simulink model "a2_sim_model"  (R2023a)
settings: Solver=ode4  StartTime=0.0  StopTime=end_time  FixedStep=dt  MaxStep=0.001  RelTol=1e-3
values from neighbouring files (symbols this model uses):
  dt = 0.001    [a3_main_scipt.m]
  IC = [x_ic, theta_ic, D_x_ic, D_theta_ic]'    [a3_main_scipt.m]
  K_Dtheta = 3    [a3_main_scipt.m]
  K_Dx = 0.01    [a3_main_scipt.m]
  K_theta = 30    [a3_main_scipt.m]
  K_x = 0.01    [a3_main_scipt.m]
libraries: simulink x2
settings Model: Creator=Adam  LastModifiedBy=Adam
settings SolverCC: AlgebraicLoopSolver=TrustRegion
settings DebuggingCC: AlgebraicLoopMsg=none  UnconnectedInputMsg=warning  UnconnectedOutputMsg=warning  UnconnectedLineMsg=warning
settings ModelReferenceCC: EnableRefExpFcnMdlSchedulingChecks=on
settings RTWCC: DLArmComputeVersion=19.05

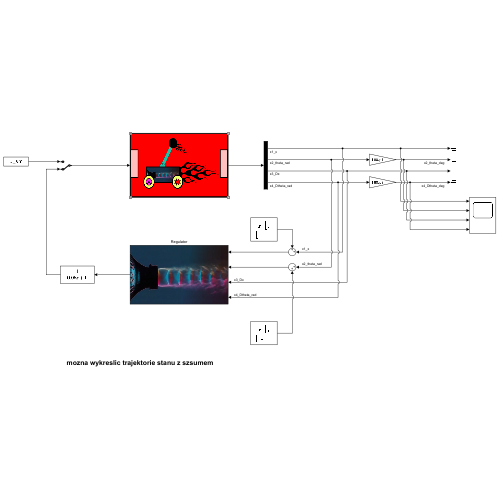
[thumbnail: Simulink's stored preview of the top-level diagram]
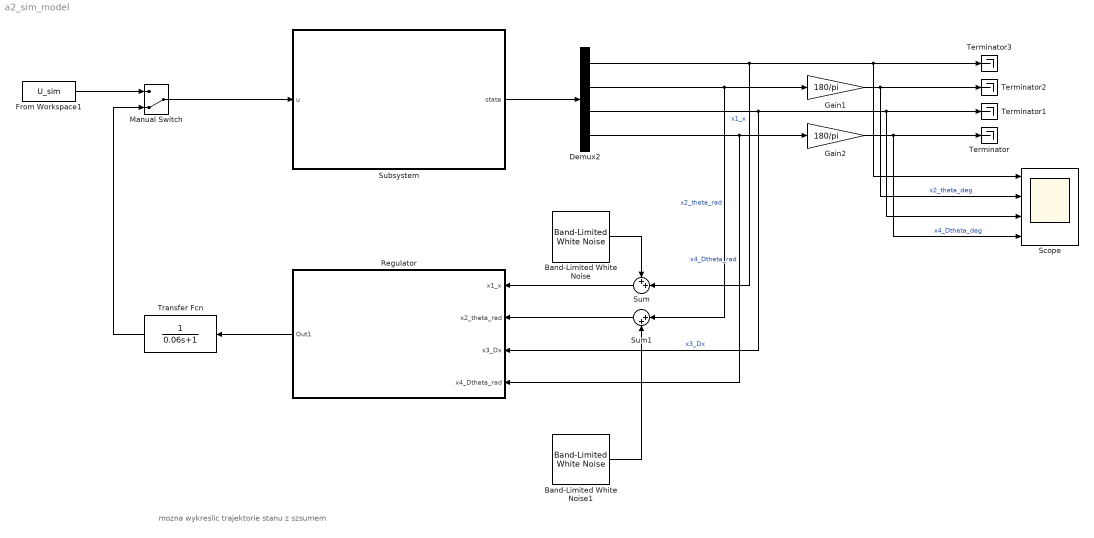
== system a2_sim_model ==
  note: mozna wykreslic trajektorie stanu z szsumem
  Band-Limited White Noise : simulink/Sources/Band-Limited White Noise  Cov=[0.0001]  Ts=0.25  seed=[23341]
  Band-Limited White Noise1 : simulink/Sources/Band-Limited White Noise  Cov=[0.0000001]  Ts=0.25  seed=[23341]
  Demux2 : Demux
  From Workspace1 : FromWorkspace  VariableName=U_sim  SampleTime=dt
  Gain1 : Gain  Gain=180/pi
  Gain2 : Gain  Gain=180/pi
  Manual Switch : ManualSwitch  CurrentSetting=0
  Regulator : Subsystem
      mask Display: image('D:\zpy_projects\wahadlo\images_drawio\wallpaper_no2.png'); % Use "Edit Image" on toolstrip to change.
  Scope : Scope  NumInputPorts=4
  Subsystem : Subsystem
      mask Display: image('D:\zpy_projects\wahadlo\images_drawio\wahadlo-wahadlo_alone_mk2.png'); % Use "Edit Image" on toolstrip to change.
  Sum : Sum  Inputs=++|
  Sum1 : Sum  Inputs=|++
  Terminator{,1..3} (4 alike) : Terminator
  Transfer Fcn : TransferFcn  Denominator=[0.06 1]
  wires:
  Gain2/1 -> Terminator/1, Scope/4  "x4_Dtheta_deg"
  Demux2/4 -> Regulator/4(x4_Dtheta_rad), Gain2/1  "x4_Dtheta_rad"
  Demux2/3 -> Regulator/3(x3_Dx), Scope/3, Terminator1/1  "x3_Dx"
  Demux2/2 -> Sum1/1, Gain1/1  "x2_theta_rad"
  Demux2/1 -> Scope/1, Terminator3/1, Sum/2  "x1_x"
  Gain1/1 -> Terminator2/1, Scope/2  "x2_theta_deg"
  From Workspace1/1 -> Manual Switch/1
  Manual Switch/1 -> Subsystem/1(u)
  Subsystem/1(state) -> Demux2/1
  Regulator/1(Out1) -> Transfer Fcn/1
  Sum/1 -> Regulator/1(x1_x)
  Band-Limited White Noise/1 -> Sum/1
  Sum1/1 -> Regulator/2(x2_theta_rad)
  Band-Limited White Noise1/1 -> Sum1/2
  Transfer Fcn/1 -> Manual Switch/2

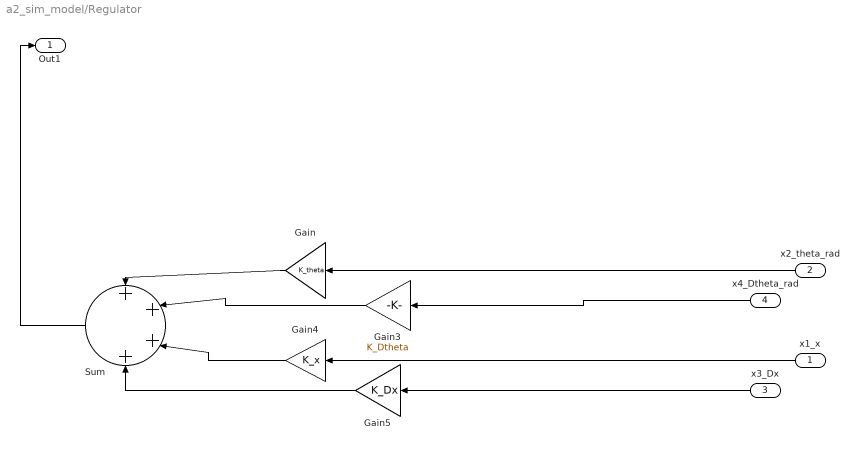
== system a2_sim_model/Regulator ==
  x1_x : Inport
  x2_theta_rad : Inport  Port=2
  x3_Dx : Inport  Port=3
  x4_Dtheta_rad : Inport  Port=4
  Gain : Gain  Gain=K_theta
  Gain3 : Gain  Gain=K_Dtheta
  Gain4 : Gain  Gain=K_x
  Gain5 : Gain  Gain=K_Dx
  Sum : Sum  Inputs=++++
  Out1 : Outport
  wires:
  x1_x/1 -> Gain4/1
  Gain4/1 -> Sum/3
  Sum/1 -> Out1/1
  x4_Dtheta_rad/1 -> Gain3/1
  Gain/1 -> Sum/1
  Gain5/1 -> Sum/4
  x2_theta_rad/1 -> Gain/1
  Gain3/1 -> Sum/2
  x3_Dx/1 -> Gain5/1

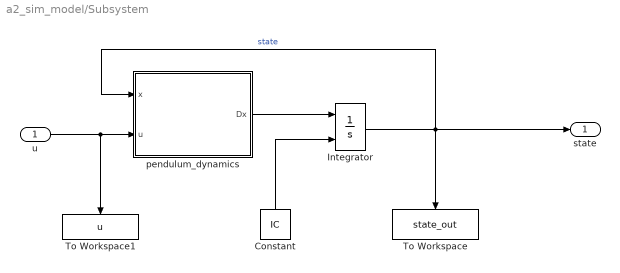
== system a2_sim_model/Subsystem ==
  u : Inport
  Constant : Constant  Value=IC
  Integrator : Integrator  InitialConditionSource=external
  To Workspace : ToWorkspace  VariableName=state_out  SaveFormat=Structure With Time  SampleTime=-1
      settings: Save2DSignal=2-D array (concatenate along first dimension)
  To Workspace1 : ToWorkspace  VariableName=u  SaveFormat=Timeseries  SampleTime=-1
  pendulum_dynamics : MATLAB Function  TreatAsAtomicUnit=on
  state : Outport
  wires:
  Integrator/1 -> state/1, pendulum_dynamics/1(x), To Workspace/1  "state"
  u/1 -> pendulum_dynamics/2(u), To Workspace1/1
  pendulum_dynamics/1(Dx) -> Integrator/1
  Constant/1 -> Integrator/2

== matlab function a2_sim_model/Subsystem/pendulum_dynamics ==
  data: x input; u input; Dx output; params parameter
function Dx = dynamika_wahadla(x, u, params)
% x : state
% u : input signal
%
% params scope: "parameters"

% State, function input: x = [x Dx theta Dtheta]'
x1 = x(1);
x2 = x(2);
x3 = x(3);
x4 = x(4);

% % Sat na x1
% if x1 >= 0.4
%     x1 = 0.4;
% elseif x1 <= -0.4
%     x1 = -0.4;
% end

% Params
% [M, mc, mp, Lp, Lc, g, b, gamma, D, alpha, mr, Mt, L, Jcm, Jt] = params.values;
M       = params(1);
mc      = params(2);
mp      = params(3);
Lp      = params(4);
Lc      = params(5);
g       = params(6);
b       = params(7);
gamma   = params(8);
D       = params(9);
alpha   = params(10);
mr      = params(11);
Mt      = params(12);
L       = params(13);
Jcm     = params(14);
Jt      = params(15);

% Equations for pendulum dynamics
den = Jt*Mt - L^2 * mr^2 * cos(x2);
ddt_x1 = x3;
ddt_x2 = x4;
ddt_x3 = ( Jt*(D*cos(alpha) + ...
           L*mr*x4^2*sin(x2) - ...
           b*x3 + u) - ...
           L*mr*cos(x2) * ( D*( L*cos(alpha-x2) + sin(alpha+pi/4) ) + ...
           L*g*mr*sin(x2) - gamma*x4 ) ) / den;

ddt_x4 = ( -L*mr*cos(x2) * (D*cos(alpha) + ...
           L*mr*x4^2*sin(x2) - ...
           b*x3 + u) + ...
           Mt * ( D*( L*cos(alpha-x2) + sin(alpha+pi/4) ) + ... 
           L*g*mr*sin(x2) - ... 
           gamma*x4 ) ) / den;

% output
Dx = [ddt_x1 ddt_x2 ddt_x3 ddt_x4]';

end
